simulink model "syt_simulink_foo"  (Simulink 7.0)
settings: Solver=ode3  StartTime=0.0  StopTime=10.0  FixedStep=0.01  RelTol=1e-3
settings Model: Creator=LAT04  LastModifiedBy=LAT04

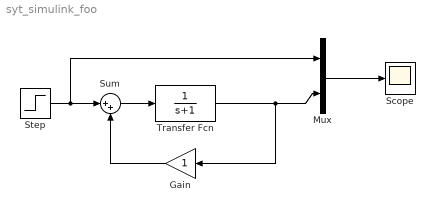
== system syt_simulink_foo ==
  Gain : Gain  Orientation=left  ParameterDataType=sfix(16)  ParameterScaling=2^0  OutDataType=sfix(16)  OutScaling=2^0
  Mux : Mux  Inputs=2
  Scope : Scope
  Step : Step  SampleTime=0
  Sum : Sum  Inputs=|++  OutDataType=sfix(16)  OutScaling=2^0
  Transfer Fcn : TransferFcn  Denominator=[1 1]
  wires:
  Mux/1 -> Scope/1
  Sum/1 -> Transfer Fcn/1
  Transfer Fcn/1 -> Gain/1, Mux/2
  Gain/1 -> Sum/2
  Step/1 -> Sum/1, Mux/1
